simulink model "Initiate_simulation_test_compatible"  (R2022a)
settings: Solver=VariableStepAuto  StartTime=0.0  StopTime=Inf  RelTol=1e-3
undefined symbols (not defined in the file or in its folder): max_deflections
libraries: aerolibanimutils x3, slpidlib x2, FlightInstruments x1, FlightSimulation_FlightMechanics_LibModelModified x1, SimulinkToXPlane11 x1
settings Model: Creator=setup  LastModifiedBy=dmgp1
settings DataIOCC: SaveState=on
settings DebuggingCC: UnconnectedInputMsg=warning  UnconnectedOutputMsg=warning  UnconnectedLineMsg=warning
settings RTWCC: DLArmComputeVersion=19.05

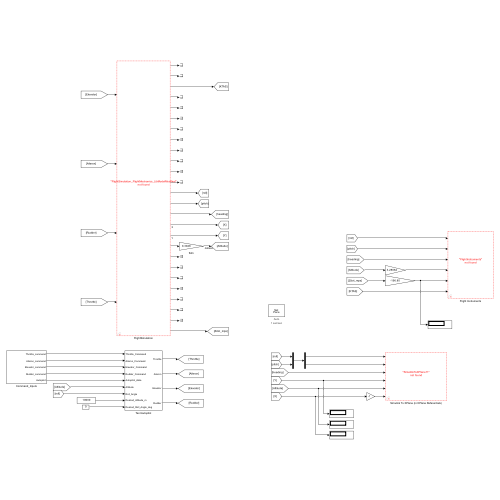
[thumbnail: Simulink's stored preview of the top-level diagram]
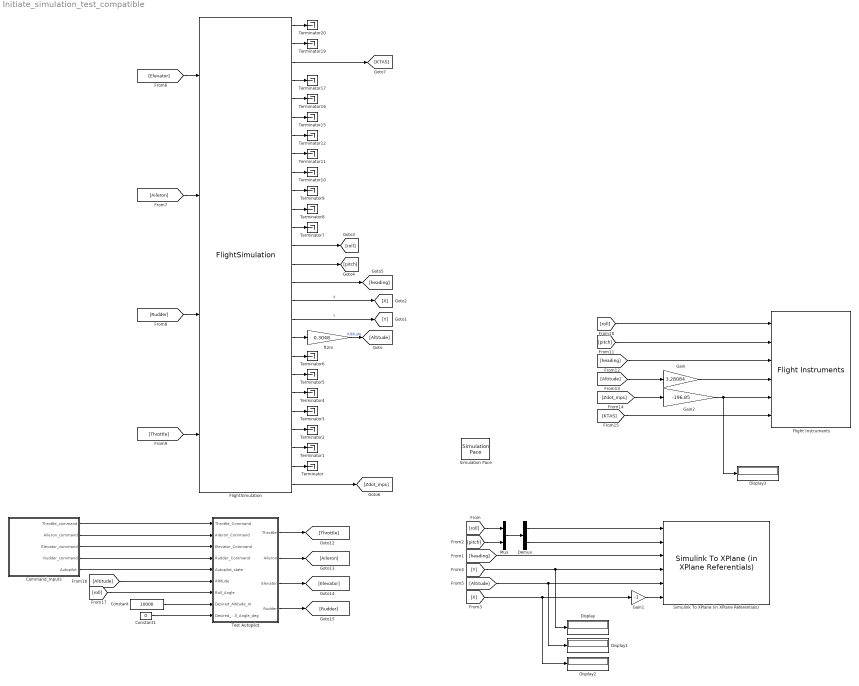
== system Initiate_simulation_test_compatible ==
  Command_Inputs : Subsystem
  Constant : Constant  Value=10000
  Constant1 : Constant  Value=0
  Demux : Demux  Outputs=2
  Display{,1..3} (4 alike) : Display
  Flight Instruments : FlightInstruments/Flight Instruments  SystemSampleTime=-1  VariantActivationTime=update diagram  Latency=0  AutoFrameSizeCalculation=off
  FlightSimulation : FlightSimulation_FlightMechanics_LibModelModified/FlightSimulation  SystemSampleTime=-1  VariantActivationTime=update diagram  Latency=0  AutoFrameSizeCalculation=off
  Gain : Gain  Gain=3.28084
  Gain1 : Gain  Gain=-1
  Gain2 : Gain  Gain=-196.85
  Mux : Mux  Inputs=2
  Simulation Pace : aerolibanimutils/Simulation Pace  SimulationPace=1  SleepMode=Auto  OutputPaceError=off  SampleTime=1/60
  Simulink To XPlane (in XPlane Referentials) : SimulinkToXPlane11/Simulink To XPlane (in XPlane Referentials)  Precision=5
  Terminator{,1..12,15..17,19..20} (18 alike) : Terminator
  Test Autopilot : Subsystem
  ft2m : Gain  Gain=0.3048
  wires:
  FlightSimulation/18 -> ft2m/1
  ft2m/1 -> [Altitude]  "Altitude"
  FlightSimulation/17 -> [Y]  "Y"
  FlightSimulation/16 -> [X]  "X"
  FlightSimulation/25 -> Terminator/1
  FlightSimulation/24 -> Terminator1/1
  FlightSimulation/22 -> Terminator3/1
  FlightSimulation/23 -> Terminator2/1
  FlightSimulation/21 -> Terminator4/1
  FlightSimulation/19 -> Terminator6/1
  FlightSimulation/20 -> Terminator5/1
  FlightSimulation/9 -> Terminator10/1
  FlightSimulation/13 -> [roll]
  FlightSimulation/14 -> [pitch]
  FlightSimulation/15 -> [heading]
  FlightSimulation/1 -> Terminator20/1
  FlightSimulation/2 -> Terminator19/1
  FlightSimulation/3 -> [KTAS]
  FlightSimulation/4 -> Terminator17/1
  FlightSimulation/5 -> Terminator16/1
  FlightSimulation/6 -> Terminator15/1
  FlightSimulation/7 -> Terminator12/1
  FlightSimulation/8 -> Terminator11/1
  [Elevator] -> FlightSimulation/1
  [Aileron] -> FlightSimulation/2
  [Rudder] -> FlightSimulation/3
  [Throttle] -> FlightSimulation/4
  FlightSimulation/10 -> Terminator9/1
  FlightSimulation/11 -> Terminator8/1
  FlightSimulation/12 -> Terminator7/1
  [heading] -> Simulink To XPlane (in XPlane Referentials)/3
  [Y] -> Simulink To XPlane (in XPlane Referentials)/4, Display/1
  [Altitude] -> Simulink To XPlane (in XPlane Referentials)/5, Display1/1
  Gain1/1 -> Simulink To XPlane (in XPlane Referentials)/6
  [X] -> Display2/1, Gain1/1
  [pitch] -> Mux/2
  [roll] -> Mux/1
  Mux/1 -> Demux/1
  Demux/1 -> Simulink To XPlane (in XPlane Referentials)/1
  Demux/2 -> Simulink To XPlane (in XPlane Referentials)/2
  [roll] -> Flight Instruments/1
  [pitch] -> Flight Instruments/2
  [heading] -> Flight Instruments/3
  Gain/1 -> Flight Instruments/4
  [Altitude] -> Gain/1
  FlightSimulation/26 -> [Zdot_mps]
  Gain2/1 -> Flight Instruments/5, Display3/1
  [Zdot_mps] -> Gain2/1
  [KTAS] -> Flight Instruments/6
  Test Autopilot/1(Throttle) -> [Throttle]
  Test Autopilot/2(Aileron) -> [Aileron]
  Test Autopilot/3(Elevator) -> [Elevator]
  Test Autopilot/4(Rudder) -> [Rudder]
  Command_Inputs/1(Throttle_command) -> Test Autopilot/1(Throttle_Command)
  Command_Inputs/2(Aileron_command) -> Test Autopilot/2(Aileron_Command)
  Command_Inputs/3(Elevator_command) -> Test Autopilot/3(Elevator_Command)
  Command_Inputs/4(Rudder_command) -> Test Autopilot/4(Rudder_Command)
  Command_Inputs/5(Autopilot) -> Test Autopilot/5(Autopilot_state)
  [Altitude] -> Test Autopilot/6(Altitude)
  [roll] -> Test Autopilot/7(Roll_Angle)
  Constant/1 -> Test Autopilot/8(Desired_Altitude_m)
  Constant1/1 -> Test Autopilot/9(Desired_Roll_Angle_deg)

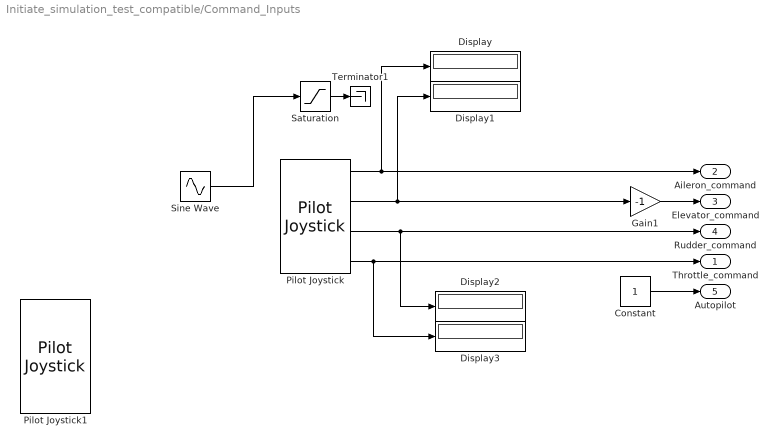
== system Initiate_simulation_test_compatible/Command_Inputs ==
  Constant : Constant
  Display{,1..3} (4 alike) : Display
  Gain1 : Gain  Gain=-1
  Pilot Joystick : aerolibanimutils/Pilot Joystick  JoystickID=Joystick1  OutputConfiguration=FourAxis  SampleTime=1/60
  Pilot Joystick1 : aerolibanimutils/Pilot Joystick  JoystickID=Joystick2  OutputConfiguration=AllOutputs  SampleTime=1/60
  Saturation : Saturate  UpperLimit=1  LowerLimit=0
  Sine Wave : Sin  SampleTime=0
  Terminator1 : Terminator
  Throttle_command : Outport
  Aileron_command : Outport  Port=2
  Elevator_command : Outport  Port=3
  Rudder_command : Outport  Port=4
  Autopilot : Outport  Port=5
  wires:
  Sine Wave/1 -> Saturation/1
  Saturation/1 -> Terminator1/1
  Pilot Joystick/4 -> Display3/1, Throttle_command/1
  Pilot Joystick/1 -> Aileron_command/1, Display/1
  Pilot Joystick/3 -> Rudder_command/1, Display2/1
  Pilot Joystick/2 -> Gain1/1, Display1/1
  Gain1/1 -> Elevator_command/1
  Constant/1 -> Autopilot/1

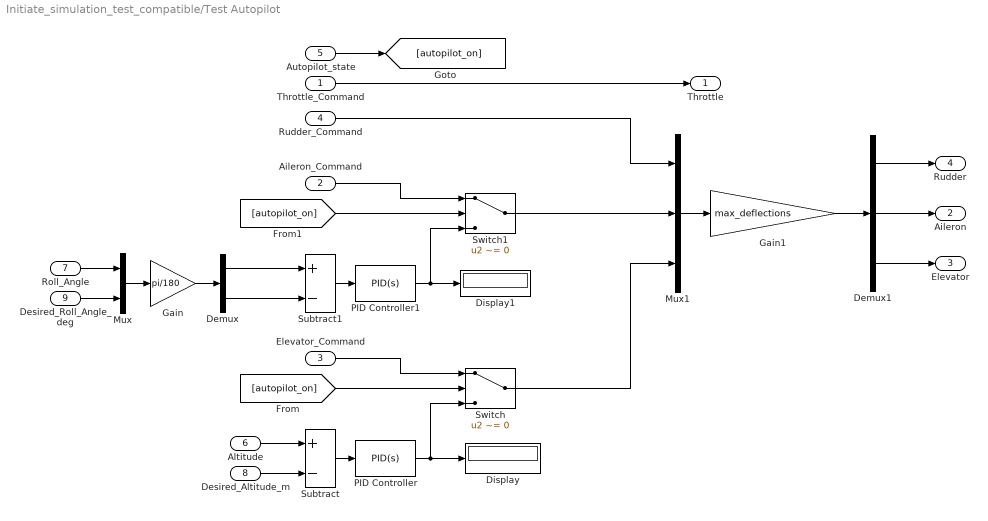
== system Initiate_simulation_test_compatible/Test Autopilot ==
  Throttle_Command : Inport
  Aileron_Command : Inport  Port=2
  Elevator_Command : Inport  Port=3
  Rudder_Command : Inport  Port=4
  Autopilot_state : Inport  Port=5
  Altitude : Inport  Port=6
  Roll_Angle : Inport  Port=7
  Desired_Altitude_m : Inport  Port=8
  Desired_Roll_Angle_deg : Inport  Port=9
  Demux : Demux  Outputs=2
  Demux1 : Demux  Outputs=3
  Display : Display
  Display1 : Display
  Gain : Gain  Gain=pi/180
  Gain1 : Gain  Gain=max_deflections  OutMin=-3  OutMax=5
  Mux : Mux  Inputs=2
  Mux1 : Mux  Inputs=3
  PID Controller : slpidlib/PID Controller  Controller=PID  Form=Parallel  TimeDomain=Continuous-time  UseExternalTs=off  SampleTime=-1  IntegratorMethod=Forward Euler  FilterMethod=Forward Euler  ControllerParametersSource=internal  P=2  I=0.5  UseKiTs=off  D=0.1  N=100  UseFilter=on  TunerSelectOption=Frequency Response Based  InitialConditionSource=internal  InitialConditionForIntegrator=0  InitialConditionForFilter=0  DifferentiatorICPrevScaledInput=0  ExternalReset=none  TrackingMode=off  Kt=1  LimitOutput=on  SatLimitsSource=internal  UpperSaturationLimit=1  LowerSaturationLimit=-1  LinearizeAsGain=on  AntiWindupMode=none  Kb=1  POutMin=[]  POutMax=[]  IOutMin=[]  IOutMax=[]  DOutMin=[]  DOutMax=[]  NOutMin=[]  NOutMax=[]  SumOutMin=[]  SumOutMax=[]  SaturationOutMin=[]  SaturationOutMax=[]  PParamMin=[]  PParamMax=[]  IParamMin=[]  IParamMax=[]  DParamMin=[]  DParamMax=[]  NParamMin=[]  NParamMax=[]  KbParamMin=[]  KbParamMax=[]  KtParamMin=[]  KtParamMax=[]  KbOutMin=[]  KbOutMax=[]  KtOutMin=[]  KtOutMax=[]  IntegratorOutMin=[]  IntegratorOutMax=[]  FilterOutMin=[]  FilterOutMax=[]  SumI1OutMin=[]  SumI1OutMax=[]  SumI2OutMin=[]  SumI2OutMax=[]  SumI3OutMin=[]  SumI3OutMax=[]  SumI4OutMin=[]  SumI4OutMax=[]  SumDOutMin=[]  SumDOutMax=[]  DifferentiatorOutMin=[]  DifferentiatorOutMax=[]  FilterDiffOutCoefMin=[]  FilterDiffOutCoefMax=[]  ReciprocalOutMin=[]  ReciprocalOutMax=[]  SumDenOutMin=[]  SumDenOutMax=[]  SumNumOutMin=[]  SumNumOutMax=[]  DivideOutMin=[]  DivideOutMax=[]  UdiffTsProdOutMin=[]  UdiffTsProdOutMax=[]  NTsProdOutMin=[]  NTsProdOutMax=[]  UintegralTsProdOutMin=[]  UintegralTsProdOutMax=[]  UngainTsProdOutMin=[]  UngainTsProdOutMax=[]  IntegratorContinuousStateAttributes=''  IntegratorStateMustResolveToSignalObject=off  IntegratorRTWStateStorageClass=Auto  FilterContinuousStateAttributes=''  FilterStateMustResolveToSignalObject=off  FilterRTWStateStorageClass=Auto  ParallelPVariant=InternalParameters  IdealPVariant=Disabled  IVariant=InternalParameters  DVariant=InternalParameters  IntegratorVariant=Continuous  SatVariant=Enabled  AWVariant=Passthrough  PCopyVariant=Disabled  TRVariant=Disabled  FdbkBlocksVariant=Forward  IdealPFdbkVariant=Disabled  SatFdbkVariant=Disabled  DerivativeFilterVariant=ContFilter  NVariant=InternalParameters  NCopyVariant=Disabled  FilterICVariant=InternalICsFilter  IntegratorICVariant=InternalICs  ExternalResetVariant=Disabled  TRSumVariant=Passthrough  SumFdbkVariant=Disabled  SumVariant=Sum_PID  TsampFilterVariant=InternalTs  TsampNgainVariant=Passthrough  TsampIntegralVariant=Disabled_SignalSpec  ExternalSaturationOutDataTypeStr=Inherit: Same as second input
  PID Controller1 : slpidlib/PID Controller  Controller=PID  Form=Parallel  TimeDomain=Continuous-time  UseExternalTs=off  SampleTime=-1  IntegratorMethod=Forward Euler  FilterMethod=Forward Euler  ControllerParametersSource=internal  P=2  I=0.5  UseKiTs=off  D=0.1  N=100  UseFilter=on  TunerSelectOption=Frequency Response Based  InitialConditionSource=internal  InitialConditionForIntegrator=0  InitialConditionForFilter=0  DifferentiatorICPrevScaledInput=0  ExternalReset=none  TrackingMode=off  Kt=1  LimitOutput=on  SatLimitsSource=internal  UpperSaturationLimit=1  LowerSaturationLimit=-1  LinearizeAsGain=on  AntiWindupMode=none  Kb=1  POutMin=[]  POutMax=[]  IOutMin=[]  IOutMax=[]  DOutMin=[]  DOutMax=[]  NOutMin=[]  NOutMax=[]  SumOutMin=[]  SumOutMax=[]  SaturationOutMin=[]  SaturationOutMax=[]  PParamMin=[]  PParamMax=[]  IParamMin=[]  IParamMax=[]  DParamMin=[]  DParamMax=[]  NParamMin=[]  NParamMax=[]  KbParamMin=[]  KbParamMax=[]  KtParamMin=[]  KtParamMax=[]  KbOutMin=[]  KbOutMax=[]  KtOutMin=[]  KtOutMax=[]  IntegratorOutMin=[]  IntegratorOutMax=[]  FilterOutMin=[]  FilterOutMax=[]  SumI1OutMin=[]  SumI1OutMax=[]  SumI2OutMin=[]  SumI2OutMax=[]  SumI3OutMin=[]  SumI3OutMax=[]  SumI4OutMin=[]  SumI4OutMax=[]  SumDOutMin=[]  SumDOutMax=[]  DifferentiatorOutMin=[]  DifferentiatorOutMax=[]  FilterDiffOutCoefMin=[]  FilterDiffOutCoefMax=[]  ReciprocalOutMin=[]  ReciprocalOutMax=[]  SumDenOutMin=[]  SumDenOutMax=[]  SumNumOutMin=[]  SumNumOutMax=[]  DivideOutMin=[]  DivideOutMax=[]  UdiffTsProdOutMin=[]  UdiffTsProdOutMax=[]  NTsProdOutMin=[]  NTsProdOutMax=[]  UintegralTsProdOutMin=[]  UintegralTsProdOutMax=[]  UngainTsProdOutMin=[]  UngainTsProdOutMax=[]  IntegratorContinuousStateAttributes=''  IntegratorStateMustResolveToSignalObject=off  IntegratorRTWStateStorageClass=Auto  FilterContinuousStateAttributes=''  FilterStateMustResolveToSignalObject=off  FilterRTWStateStorageClass=Auto  ParallelPVariant=InternalParameters  IdealPVariant=Disabled  IVariant=InternalParameters  DVariant=InternalParameters  IntegratorVariant=Continuous  SatVariant=Enabled  AWVariant=Passthrough  PCopyVariant=Disabled  TRVariant=Disabled  FdbkBlocksVariant=Forward  IdealPFdbkVariant=Disabled  SatFdbkVariant=Disabled  DerivativeFilterVariant=ContFilter  NVariant=InternalParameters  NCopyVariant=Disabled  FilterICVariant=InternalICsFilter  IntegratorICVariant=InternalICs  ExternalResetVariant=Disabled  TRSumVariant=Passthrough  SumFdbkVariant=Disabled  SumVariant=Sum_PID  TsampFilterVariant=InternalTs  TsampNgainVariant=Passthrough  TsampIntegralVariant=Disabled_SignalSpec  ExternalSaturationOutDataTypeStr=Inherit: Same as second input
  Subtract : Sum  Inputs=+-
  Subtract1 : Sum  Inputs=+-
  Switch : Switch  Criteria=u2 ~= 0  SaturateOnIntegerOverflow=off  InputSameDT=off
  Switch1 : Switch  Criteria=u2 ~= 0  SaturateOnIntegerOverflow=off  InputSameDT=off
  Throttle : Outport
  Aileron : Outport  Port=2
  Elevator : Outport  Port=3
  Rudder : Outport  Port=4
  wires:
  Throttle_Command/1 -> Throttle/1
  Elevator_Command/1 -> Switch/1
  Altitude/1 -> Subtract/1
  Desired_Altitude_m/1 -> Subtract/2
  Subtract/1 -> PID Controller/1
  PID Controller/1 -> Switch/3, Display/1
  Autopilot_state/1 -> [autopilot_on]
  [autopilot_on] -> Switch/2
  PID Controller1/1 -> Display1/1, Switch1/3
  Aileron_Command/1 -> Switch1/1
  [autopilot_on] -> Switch1/2
  Subtract1/1 -> PID Controller1/1
  Desired_Roll_Angle_deg/1 -> Mux/2
  Roll_Angle/1 -> Mux/1
  Mux/1 -> Gain/1
  Demux/1 -> Subtract1/1
  Demux/2 -> Subtract1/2
  Gain/1 -> Demux/1
  Switch1/1 -> Mux1/2
  Rudder_Command/1 -> Mux1/1
  Switch/1 -> Mux1/3
  Mux1/1 -> Gain1/1
  Gain1/1 -> Demux1/1
  Demux1/2 -> Aileron/1
  Demux1/1 -> Rudder/1
  Demux1/3 -> Elevator/1
